simulink model "firefighting_drone_2"  (R2022b)
settings: Solver=FixedStepAuto  StartTime=0.0  StopTime=80  FixedStep=0.1  RelTol=1e-3
(part 3 of 4)

== system firefighting_drone_2/Search for Fire/Seaerch-fire/Search5/Move Arm1 ==
  Speed : Inport
  Starting Angle : Inport  Port=2
  Desired Angle : Inport  Port=3
  If : If
  If Action Subsystem : Subsystem  TreatAsAtomicUnit=on
  If Action Subsystem1 : Subsystem  TreatAsAtomicUnit=on
  Integrator1 : Integrator
  Scope : Scope
  Scope1 : Scope
  Subsystem : Subsystem
  Sum1 : Sum  Inputs=|++
  Sum2 : Sum  Inputs=|+-
  Sum3 : Sum  Inputs=|-+
  Switch : Switch  Criteria=u2 ~= 0  SaturateOnIntegerOverflow=off  InputSameDT=off
  Out1 : Outport  VectorParamsAs1DForOutWhenUnconnected=off
  Done : Outport  Port=2  VectorParamsAs1DForOutWhenUnconnected=off
  wires:
  Speed/1 -> Integrator1/1
  If Action Subsystem/1(Out1) -> Switch/3
  Sum2/1 -> If/1
  If/2 -> If Action Subsystem1/Action
  Starting Angle/1 -> Sum2/2, Sum3/2, Sum1/2
  Desired Angle/1 -> Scope1/1, Subsystem/1(Desired Angle), Sum2/1
  If Action Subsystem1/1(Out1) -> Switch/1, Switch/2
  If/1 -> If Action Subsystem/Action
  Integrator1/1 -> Sum1/1, Sum3/1
  Sum3/1 -> If Action Subsystem1/1(In1)
  Sum1/1 -> If Action Subsystem/1(In1)
  Switch/1 -> Subsystem/2(Current Angle)
  Subsystem/1(Out1) -> Scope/1, Out1/1
  Subsystem/2(Done) -> Done/1

== system firefighting_drone_2/Search for Fire/Seaerch-fire/Search5/Move Arm2 ==
  Speed : Inport
  Starting Angle : Inport  Port=2
  Desired Angle : Inport  Port=3
  If : If
  If Action Subsystem : Subsystem  TreatAsAtomicUnit=on
  If Action Subsystem1 : Subsystem  TreatAsAtomicUnit=on
  Integrator1 : Integrator
  Scope : Scope
  Subsystem : Subsystem
  Sum1 : Sum  Inputs=|++
  Sum2 : Sum  Inputs=|+-
  Sum3 : Sum  Inputs=|-+
  Switch : Switch  Criteria=u2 ~= 0  SaturateOnIntegerOverflow=off  InputSameDT=off
  Out1 : Outport  VectorParamsAs1DForOutWhenUnconnected=off
  Done : Outport  Port=2  VectorParamsAs1DForOutWhenUnconnected=off
  wires:
  Speed/1 -> Integrator1/1
  If Action Subsystem/1(Out1) -> Switch/3
  Sum2/1 -> If/1
  If/2 -> If Action Subsystem1/Action
  Starting Angle/1 -> Sum2/2, Sum3/2, Sum1/2
  Desired Angle/1 -> Subsystem/1(Desired Angle), Sum2/1
  If Action Subsystem1/1(Out1) -> Switch/1, Switch/2
  If/1 -> If Action Subsystem/Action
  Integrator1/1 -> Sum1/1, Sum3/1
  Sum3/1 -> If Action Subsystem1/1(In1)
  Sum1/1 -> If Action Subsystem/1(In1)
  Switch/1 -> Subsystem/2(Current Angle)
  Subsystem/1(Out1) -> Scope/1, Out1/1
  Subsystem/2(Done) -> Done/1

== system firefighting_drone_2/Search for Fire/Seaerch-fire/Search5/Move Arm3 ==
  Speed : Inport
  Starting Angle : Inport  Port=2
  Desired Angle : Inport  Port=3
  If : If
  If Action Subsystem : Subsystem  TreatAsAtomicUnit=on
  If Action Subsystem1 : Subsystem  TreatAsAtomicUnit=on
  Integrator1 : Integrator
  Scope : Scope
  Subsystem : Subsystem
  Sum1 : Sum  Inputs=|++
  Sum2 : Sum  Inputs=|+-
  Sum3 : Sum  Inputs=|-+
  Switch : Switch  Criteria=u2 ~= 0  SaturateOnIntegerOverflow=off  InputSameDT=off
  Out1 : Outport  VectorParamsAs1DForOutWhenUnconnected=off
  Done : Outport  Port=2  VectorParamsAs1DForOutWhenUnconnected=off
  wires:
  Speed/1 -> Integrator1/1
  If Action Subsystem/1(Out1) -> Switch/3
  Sum2/1 -> If/1
  If/2 -> If Action Subsystem1/Action
  Starting Angle/1 -> Sum2/2, Sum3/2, Sum1/2
  Desired Angle/1 -> Subsystem/1(Desired Angle), Sum2/1
  If Action Subsystem1/1(Out1) -> Switch/1, Switch/2
  If/1 -> If Action Subsystem/Action
  Integrator1/1 -> Sum1/1, Sum3/1
  Sum3/1 -> If Action Subsystem1/1(In1)
  Sum1/1 -> If Action Subsystem/1(In1)
  Switch/1 -> Subsystem/2(Current Angle)
  Subsystem/1(Out1) -> Scope/1, Out1/1
  Subsystem/2(Done) -> Done/1

== system firefighting_drone_2/Search for Fire/Seaerch-fire/Search6/Move Arm1 ==
  Speed : Inport
  Starting Angle : Inport  Port=2
  Desired Angle : Inport  Port=3
  If : If
  If Action Subsystem : Subsystem  TreatAsAtomicUnit=on
  If Action Subsystem1 : Subsystem  TreatAsAtomicUnit=on
  Integrator1 : Integrator
  Scope : Scope
  Scope1 : Scope
  Subsystem : Subsystem
  Sum1 : Sum  Inputs=|++
  Sum2 : Sum  Inputs=|+-
  Sum3 : Sum  Inputs=|-+
  Switch : Switch  Criteria=u2 ~= 0  SaturateOnIntegerOverflow=off  InputSameDT=off
  Out1 : Outport  VectorParamsAs1DForOutWhenUnconnected=off
  Done : Outport  Port=2  VectorParamsAs1DForOutWhenUnconnected=off
  wires:
  Speed/1 -> Integrator1/1
  If Action Subsystem/1(Out1) -> Switch/3
  Sum2/1 -> If/1
  If/2 -> If Action Subsystem1/Action
  Starting Angle/1 -> Sum2/2, Sum3/2, Sum1/2
  Desired Angle/1 -> Scope1/1, Subsystem/1(Desired Angle), Sum2/1
  If Action Subsystem1/1(Out1) -> Switch/1, Switch/2
  If/1 -> If Action Subsystem/Action
  Integrator1/1 -> Sum1/1, Sum3/1
  Sum3/1 -> If Action Subsystem1/1(In1)
  Sum1/1 -> If Action Subsystem/1(In1)
  Switch/1 -> Subsystem/2(Current Angle)
  Subsystem/1(Out1) -> Scope/1, Out1/1
  Subsystem/2(Done) -> Done/1

== system firefighting_drone_2/Search for Fire/Seaerch-fire/Search6/Move Arm2 ==
  Speed : Inport
  Starting Angle : Inport  Port=2
  Desired Angle : Inport  Port=3
  If : If
  If Action Subsystem : Subsystem  TreatAsAtomicUnit=on
  If Action Subsystem1 : Subsystem  TreatAsAtomicUnit=on
  Integrator1 : Integrator
  Scope : Scope
  Subsystem : Subsystem
  Sum1 : Sum  Inputs=|++
  Sum2 : Sum  Inputs=|+-
  Sum3 : Sum  Inputs=|-+
  Switch : Switch  Criteria=u2 ~= 0  SaturateOnIntegerOverflow=off  InputSameDT=off
  Out1 : Outport  VectorParamsAs1DForOutWhenUnconnected=off
  Done : Outport  Port=2  VectorParamsAs1DForOutWhenUnconnected=off
  wires:
  Speed/1 -> Integrator1/1
  If Action Subsystem/1(Out1) -> Switch/3
  Sum2/1 -> If/1
  If/2 -> If Action Subsystem1/Action
  Starting Angle/1 -> Sum2/2, Sum3/2, Sum1/2
  Desired Angle/1 -> Subsystem/1(Desired Angle), Sum2/1
  If Action Subsystem1/1(Out1) -> Switch/1, Switch/2
  If/1 -> If Action Subsystem/Action
  Integrator1/1 -> Sum1/1, Sum3/1
  Sum3/1 -> If Action Subsystem1/1(In1)
  Sum1/1 -> If Action Subsystem/1(In1)
  Switch/1 -> Subsystem/2(Current Angle)
  Subsystem/1(Out1) -> Scope/1, Out1/1
  Subsystem/2(Done) -> Done/1

== system firefighting_drone_2/Search for Fire/Seaerch-fire/Search6/Move Arm3 ==
  Speed : Inport
  Starting Angle : Inport  Port=2
  Desired Angle : Inport  Port=3
  If : If
  If Action Subsystem : Subsystem  TreatAsAtomicUnit=on
  If Action Subsystem1 : Subsystem  TreatAsAtomicUnit=on
  Integrator1 : Integrator
  Scope : Scope
  Subsystem : Subsystem
  Sum1 : Sum  Inputs=|++
  Sum2 : Sum  Inputs=|+-
  Sum3 : Sum  Inputs=|-+
  Switch : Switch  Criteria=u2 ~= 0  SaturateOnIntegerOverflow=off  InputSameDT=off
  Out1 : Outport  VectorParamsAs1DForOutWhenUnconnected=off
  Done : Outport  Port=2  VectorParamsAs1DForOutWhenUnconnected=off
  wires:
  Speed/1 -> Integrator1/1
  If Action Subsystem/1(Out1) -> Switch/3
  Sum2/1 -> If/1
  If/2 -> If Action Subsystem1/Action
  Starting Angle/1 -> Sum2/2, Sum3/2, Sum1/2
  Desired Angle/1 -> Subsystem/1(Desired Angle), Sum2/1
  If Action Subsystem1/1(Out1) -> Switch/1, Switch/2
  If/1 -> If Action Subsystem/Action
  Integrator1/1 -> Sum1/1, Sum3/1
  Sum3/1 -> If Action Subsystem1/1(In1)
  Sum1/1 -> If Action Subsystem/1(In1)
  Switch/1 -> Subsystem/2(Current Angle)
  Subsystem/1(Out1) -> Scope/1, Out1/1
  Subsystem/2(Done) -> Done/1

== system firefighting_drone_2/Search for Fire/Seaerch-fire/Search7/Move Arm1 ==
  Speed : Inport
  Starting Angle : Inport  Port=2
  Desired Angle : Inport  Port=3
  If : If
  If Action Subsystem : Subsystem  TreatAsAtomicUnit=on
  If Action Subsystem1 : Subsystem  TreatAsAtomicUnit=on
  Integrator1 : Integrator
  Scope : Scope
  Scope1 : Scope
  Subsystem : Subsystem
  Sum1 : Sum  Inputs=|++
  Sum2 : Sum  Inputs=|+-
  Sum3 : Sum  Inputs=|-+
  Switch : Switch  Criteria=u2 ~= 0  SaturateOnIntegerOverflow=off  InputSameDT=off
  Out1 : Outport  VectorParamsAs1DForOutWhenUnconnected=off
  Done : Outport  Port=2  VectorParamsAs1DForOutWhenUnconnected=off
  wires:
  Speed/1 -> Integrator1/1
  If Action Subsystem/1(Out1) -> Switch/3
  Sum2/1 -> If/1
  If/2 -> If Action Subsystem1/Action
  Starting Angle/1 -> Sum2/2, Sum3/2, Sum1/2
  Desired Angle/1 -> Scope1/1, Subsystem/1(Desired Angle), Sum2/1
  If Action Subsystem1/1(Out1) -> Switch/1, Switch/2
  If/1 -> If Action Subsystem/Action
  Integrator1/1 -> Sum1/1, Sum3/1
  Sum3/1 -> If Action Subsystem1/1(In1)
  Sum1/1 -> If Action Subsystem/1(In1)
  Switch/1 -> Subsystem/2(Current Angle)
  Subsystem/1(Out1) -> Scope/1, Out1/1
  Subsystem/2(Done) -> Done/1

== system firefighting_drone_2/Search for Fire/Seaerch-fire/Search7/Move Arm2 ==
  Speed : Inport
  Starting Angle : Inport  Port=2
  Desired Angle : Inport  Port=3
  If : If
  If Action Subsystem : Subsystem  TreatAsAtomicUnit=on
  If Action Subsystem1 : Subsystem  TreatAsAtomicUnit=on
  Integrator1 : Integrator
  Scope : Scope
  Subsystem : Subsystem
  Sum1 : Sum  Inputs=|++
  Sum2 : Sum  Inputs=|+-
  Sum3 : Sum  Inputs=|-+
  Switch : Switch  Criteria=u2 ~= 0  SaturateOnIntegerOverflow=off  InputSameDT=off
  Out1 : Outport  VectorParamsAs1DForOutWhenUnconnected=off
  Done : Outport  Port=2  VectorParamsAs1DForOutWhenUnconnected=off
  wires:
  Speed/1 -> Integrator1/1
  If Action Subsystem/1(Out1) -> Switch/3
  Sum2/1 -> If/1
  If/2 -> If Action Subsystem1/Action
  Starting Angle/1 -> Sum2/2, Sum3/2, Sum1/2
  Desired Angle/1 -> Subsystem/1(Desired Angle), Sum2/1
  If Action Subsystem1/1(Out1) -> Switch/1, Switch/2
  If/1 -> If Action Subsystem/Action
  Integrator1/1 -> Sum1/1, Sum3/1
  Sum3/1 -> If Action Subsystem1/1(In1)
  Sum1/1 -> If Action Subsystem/1(In1)
  Switch/1 -> Subsystem/2(Current Angle)
  Subsystem/1(Out1) -> Scope/1, Out1/1
  Subsystem/2(Done) -> Done/1

== system firefighting_drone_2/Search for Fire/Seaerch-fire/Search7/Move Arm3 ==
  Speed : Inport
  Starting Angle : Inport  Port=2
  Desired Angle : Inport  Port=3
  If : If
  If Action Subsystem : Subsystem  TreatAsAtomicUnit=on
  If Action Subsystem1 : Subsystem  TreatAsAtomicUnit=on
  Integrator1 : Integrator
  Scope : Scope
  Subsystem : Subsystem
  Sum1 : Sum  Inputs=|++
  Sum2 : Sum  Inputs=|+-
  Sum3 : Sum  Inputs=|-+
  Switch : Switch  Criteria=u2 ~= 0  SaturateOnIntegerOverflow=off  InputSameDT=off
  Out1 : Outport  VectorParamsAs1DForOutWhenUnconnected=off
  Done : Outport  Port=2  VectorParamsAs1DForOutWhenUnconnected=off
  wires:
  Speed/1 -> Integrator1/1
  If Action Subsystem/1(Out1) -> Switch/3
  Sum2/1 -> If/1
  If/2 -> If Action Subsystem1/Action
  Starting Angle/1 -> Sum2/2, Sum3/2, Sum1/2
  Desired Angle/1 -> Subsystem/1(Desired Angle), Sum2/1
  If Action Subsystem1/1(Out1) -> Switch/1, Switch/2
  If/1 -> If Action Subsystem/Action
  Integrator1/1 -> Sum1/1, Sum3/1
  Sum3/1 -> If Action Subsystem1/1(In1)
  Sum1/1 -> If Action Subsystem/1(In1)
  Switch/1 -> Subsystem/2(Current Angle)
  Subsystem/1(Out1) -> Scope/1, Out1/1
  Subsystem/2(Done) -> Done/1

== system firefighting_drone_2/Search for Fire/Seaerch-fire/Search8/Move Arm1 ==
  Speed : Inport
  Starting Angle : Inport  Port=2
  Desired Angle : Inport  Port=3
  If : If
  If Action Subsystem : Subsystem  TreatAsAtomicUnit=on
  If Action Subsystem1 : Subsystem  TreatAsAtomicUnit=on
  Integrator1 : Integrator
  Scope : Scope
  Scope1 : Scope
  Subsystem : Subsystem
  Sum1 : Sum  Inputs=|++
  Sum2 : Sum  Inputs=|+-
  Sum3 : Sum  Inputs=|-+
  Switch : Switch  Criteria=u2 ~= 0  SaturateOnIntegerOverflow=off  InputSameDT=off
  Out1 : Outport  VectorParamsAs1DForOutWhenUnconnected=off
  Done : Outport  Port=2  VectorParamsAs1DForOutWhenUnconnected=off
  wires:
  Speed/1 -> Integrator1/1
  If Action Subsystem/1(Out1) -> Switch/3
  Sum2/1 -> If/1
  If/2 -> If Action Subsystem1/Action
  Starting Angle/1 -> Sum2/2, Sum3/2, Sum1/2
  Desired Angle/1 -> Scope1/1, Subsystem/1(Desired Angle), Sum2/1
  If Action Subsystem1/1(Out1) -> Switch/1, Switch/2
  If/1 -> If Action Subsystem/Action
  Integrator1/1 -> Sum1/1, Sum3/1
  Sum3/1 -> If Action Subsystem1/1(In1)
  Sum1/1 -> If Action Subsystem/1(In1)
  Switch/1 -> Subsystem/2(Current Angle)
  Subsystem/1(Out1) -> Scope/1, Out1/1
  Subsystem/2(Done) -> Done/1

== system firefighting_drone_2/Search for Fire/Seaerch-fire/Search8/Move Arm2 ==
  Speed : Inport
  Starting Angle : Inport  Port=2
  Desired Angle : Inport  Port=3
  If : If
  If Action Subsystem : Subsystem  TreatAsAtomicUnit=on
  If Action Subsystem1 : Subsystem  TreatAsAtomicUnit=on
  Integrator1 : Integrator
  Scope : Scope
  Subsystem : Subsystem
  Sum1 : Sum  Inputs=|++
  Sum2 : Sum  Inputs=|+-
  Sum3 : Sum  Inputs=|-+
  Switch : Switch  Criteria=u2 ~= 0  SaturateOnIntegerOverflow=off  InputSameDT=off
  Out1 : Outport  VectorParamsAs1DForOutWhenUnconnected=off
  Done : Outport  Port=2  VectorParamsAs1DForOutWhenUnconnected=off
  wires:
  Speed/1 -> Integrator1/1
  If Action Subsystem/1(Out1) -> Switch/3
  Sum2/1 -> If/1
  If/2 -> If Action Subsystem1/Action
  Starting Angle/1 -> Sum2/2, Sum3/2, Sum1/2
  Desired Angle/1 -> Subsystem/1(Desired Angle), Sum2/1
  If Action Subsystem1/1(Out1) -> Switch/1, Switch/2
  If/1 -> If Action Subsystem/Action
  Integrator1/1 -> Sum1/1, Sum3/1
  Sum3/1 -> If Action Subsystem1/1(In1)
  Sum1/1 -> If Action Subsystem/1(In1)
  Switch/1 -> Subsystem/2(Current Angle)
  Subsystem/1(Out1) -> Scope/1, Out1/1
  Subsystem/2(Done) -> Done/1

== system firefighting_drone_2/Search for Fire/Seaerch-fire/Search8/Move Arm3 ==
  Speed : Inport
  Starting Angle : Inport  Port=2
  Desired Angle : Inport  Port=3
  If : If
  If Action Subsystem : Subsystem  TreatAsAtomicUnit=on
  If Action Subsystem1 : Subsystem  TreatAsAtomicUnit=on
  Integrator1 : Integrator
  Scope : Scope
  Subsystem : Subsystem
  Sum1 : Sum  Inputs=|++
  Sum2 : Sum  Inputs=|+-
  Sum3 : Sum  Inputs=|-+
  Switch : Switch  Criteria=u2 ~= 0  SaturateOnIntegerOverflow=off  InputSameDT=off
  Out1 : Outport  VectorParamsAs1DForOutWhenUnconnected=off
  Done : Outport  Port=2  VectorParamsAs1DForOutWhenUnconnected=off
  wires:
  Speed/1 -> Integrator1/1
  If Action Subsystem/1(Out1) -> Switch/3
  Sum2/1 -> If/1
  If/2 -> If Action Subsystem1/Action
  Starting Angle/1 -> Sum2/2, Sum3/2, Sum1/2
  Desired Angle/1 -> Subsystem/1(Desired Angle), Sum2/1
  If Action Subsystem1/1(Out1) -> Switch/1, Switch/2
  If/1 -> If Action Subsystem/Action
  Integrator1/1 -> Sum1/1, Sum3/1
  Sum3/1 -> If Action Subsystem1/1(In1)
  Sum1/1 -> If Action Subsystem/1(In1)
  Switch/1 -> Subsystem/2(Current Angle)
  Subsystem/1(Out1) -> Scope/1, Out1/1
  Subsystem/2(Done) -> Done/1

== system firefighting_drone_2/Search for Fire/Seaerch-fire/Search9/Move Arm1 ==
  Speed : Inport
  Starting Angle : Inport  Port=2
  Desired Angle : Inport  Port=3
  If : If
  If Action Subsystem : Subsystem  TreatAsAtomicUnit=on
  If Action Subsystem1 : Subsystem  TreatAsAtomicUnit=on
  Integrator1 : Integrator
  Scope : Scope
  Scope1 : Scope
  Subsystem : Subsystem
  Sum1 : Sum  Inputs=|++
  Sum2 : Sum  Inputs=|+-
  Sum3 : Sum  Inputs=|-+
  Switch : Switch  Criteria=u2 ~= 0  SaturateOnIntegerOverflow=off  InputSameDT=off
  Out1 : Outport  VectorParamsAs1DForOutWhenUnconnected=off
  Done : Outport  Port=2  VectorParamsAs1DForOutWhenUnconnected=off
  wires:
  Speed/1 -> Integrator1/1
  If Action Subsystem/1(Out1) -> Switch/3
  Sum2/1 -> If/1
  If/2 -> If Action Subsystem1/Action
  Starting Angle/1 -> Sum2/2, Sum3/2, Sum1/2
  Desired Angle/1 -> Scope1/1, Subsystem/1(Desired Angle), Sum2/1
  If Action Subsystem1/1(Out1) -> Switch/1, Switch/2
  If/1 -> If Action Subsystem/Action
  Integrator1/1 -> Sum1/1, Sum3/1
  Sum3/1 -> If Action Subsystem1/1(In1)
  Sum1/1 -> If Action Subsystem/1(In1)
  Switch/1 -> Subsystem/2(Current Angle)
  Subsystem/1(Out1) -> Scope/1, Out1/1
  Subsystem/2(Done) -> Done/1

== system firefighting_drone_2/Search for Fire/Seaerch-fire/Search9/Move Arm2 ==
  Speed : Inport
  Starting Angle : Inport  Port=2
  Desired Angle : Inport  Port=3
  If : If
  If Action Subsystem : Subsystem  TreatAsAtomicUnit=on
  If Action Subsystem1 : Subsystem  TreatAsAtomicUnit=on
  Integrator1 : Integrator
  Scope : Scope
  Subsystem : Subsystem
  Sum1 : Sum  Inputs=|++
  Sum2 : Sum  Inputs=|+-
  Sum3 : Sum  Inputs=|-+
  Switch : Switch  Criteria=u2 ~= 0  SaturateOnIntegerOverflow=off  InputSameDT=off
  Out1 : Outport  VectorParamsAs1DForOutWhenUnconnected=off
  Done : Outport  Port=2  VectorParamsAs1DForOutWhenUnconnected=off
  wires:
  Speed/1 -> Integrator1/1
  If Action Subsystem/1(Out1) -> Switch/3
  Sum2/1 -> If/1
  If/2 -> If Action Subsystem1/Action
  Starting Angle/1 -> Sum2/2, Sum3/2, Sum1/2
  Desired Angle/1 -> Subsystem/1(Desired Angle), Sum2/1
  If Action Subsystem1/1(Out1) -> Switch/1, Switch/2
  If/1 -> If Action Subsystem/Action
  Integrator1/1 -> Sum1/1, Sum3/1
  Sum3/1 -> If Action Subsystem1/1(In1)
  Sum1/1 -> If Action Subsystem/1(In1)
  Switch/1 -> Subsystem/2(Current Angle)
  Subsystem/1(Out1) -> Scope/1, Out1/1
  Subsystem/2(Done) -> Done/1

== system firefighting_drone_2/Search for Fire/Seaerch-fire/Search9/Move Arm3 ==
  Speed : Inport
  Starting Angle : Inport  Port=2
  Desired Angle : Inport  Port=3
  If : If
  If Action Subsystem : Subsystem  TreatAsAtomicUnit=on
  If Action Subsystem1 : Subsystem  TreatAsAtomicUnit=on
  Integrator1 : Integrator
  Scope : Scope
  Subsystem : Subsystem
  Sum1 : Sum  Inputs=|++
  Sum2 : Sum  Inputs=|+-
  Sum3 : Sum  Inputs=|-+
  Switch : Switch  Criteria=u2 ~= 0  SaturateOnIntegerOverflow=off  InputSameDT=off
  Out1 : Outport  VectorParamsAs1DForOutWhenUnconnected=off
  Done : Outport  Port=2  VectorParamsAs1DForOutWhenUnconnected=off
  wires:
  Speed/1 -> Integrator1/1
  If Action Subsystem/1(Out1) -> Switch/3
  Sum2/1 -> If/1
  If/2 -> If Action Subsystem1/Action
  Starting Angle/1 -> Sum2/2, Sum3/2, Sum1/2
  Desired Angle/1 -> Subsystem/1(Desired Angle), Sum2/1
  If Action Subsystem1/1(Out1) -> Switch/1, Switch/2
  If/1 -> If Action Subsystem/Action
  Integrator1/1 -> Sum1/1, Sum3/1
  Sum3/1 -> If Action Subsystem1/1(In1)
  Sum1/1 -> If Action Subsystem/1(In1)
  Switch/1 -> Subsystem/2(Current Angle)
  Subsystem/1(Out1) -> Scope/1, Out1/1
  Subsystem/2(Done) -> Done/1

== system firefighting_drone_2/Search for Fire/Seaerch-fire/Search/Move Arm1/If Action Subsystem ==
  In1 : Inport
  Action Port : ActionPort  ActionPortLabel=if(u1 > 0)
  Out1 : Outport  VectorParamsAs1DForOutWhenUnconnected=off
  wires:
  In1/1 -> Out1/1

== system firefighting_drone_2/Search for Fire/Seaerch-fire/Search/Move Arm1/If Action Subsystem1 ==
  In1 : Inport
  Action Port : ActionPort  ActionPortLabel=else
  Out1 : Outport  VectorParamsAs1DForOutWhenUnconnected=off
  wires:
  In1/1 -> Out1/1

== system firefighting_drone_2/Search for Fire/Seaerch-fire/Search/Move Arm1/Subsystem ==
  Desired Angle : Inport
  Current Angle : Inport  Port=2
  Abs : Abs  SaturateOnIntegerOverflow=off
  Constant : Constant
  Logical Operator : Logic  Operator=OR  AllPortsSameDT=off  OutDataTypeStr=boolean
  Memory : Memory
  Relational Operator : RelationalOperator  Operator=<=  OutDataTypeStr=boolean  RndMeth=Simplest  InputSameDT=off
  Sum : Sum  Inputs=|+-
  Switch1 : Switch  Criteria=u2 > Threshold  SaturateOnIntegerOverflow=off  InputSameDT=off
  Out1 : Outport  VectorParamsAs1DForOutWhenUnconnected=off
  Done : Outport  Port=2  VectorParamsAs1DForOutWhenUnconnected=off
  wires:
  Switch1/1 -> Out1/1
  Desired Angle/1 -> Sum/1, Switch1/1
  Current Angle/1 -> Switch1/3, Sum/2
  Sum/1 -> Abs/1
  Abs/1 -> Relational Operator/1
  Constant/1 -> Relational Operator/2
  Relational Operator/1 -> Logical Operator/2
  Logical Operator/1 -> Memory/1, Done/1, Switch1/2
  Memory/1 -> Logical Operator/1

== system firefighting_drone_2/Search for Fire/Seaerch-fire/Search/Move Arm2/If Action Subsystem ==
  In1 : Inport
  Action Port : ActionPort  ActionPortLabel=if(u1 > 0)
  Out1 : Outport  VectorParamsAs1DForOutWhenUnconnected=off
  wires:
  In1/1 -> Out1/1

== system firefighting_drone_2/Search for Fire/Seaerch-fire/Search/Move Arm2/If Action Subsystem1 ==
  In1 : Inport
  Action Port : ActionPort  ActionPortLabel=else
  Out1 : Outport  VectorParamsAs1DForOutWhenUnconnected=off
  wires:
  In1/1 -> Out1/1

== system firefighting_drone_2/Search for Fire/Seaerch-fire/Search/Move Arm2/Subsystem ==
  Desired Angle : Inport
  Current Angle : Inport  Port=2
  Abs : Abs  SaturateOnIntegerOverflow=off
  Constant : Constant
  Logical Operator : Logic  Operator=OR  AllPortsSameDT=off  OutDataTypeStr=boolean
  Memory : Memory
  Relational Operator : RelationalOperator  Operator=<=  OutDataTypeStr=boolean  RndMeth=Simplest  InputSameDT=off
  Sum : Sum  Inputs=|+-
  Switch1 : Switch  Criteria=u2 > Threshold  SaturateOnIntegerOverflow=off  InputSameDT=off
  Out1 : Outport  VectorParamsAs1DForOutWhenUnconnected=off
  Done : Outport  Port=2  VectorParamsAs1DForOutWhenUnconnected=off
  wires:
  Switch1/1 -> Out1/1
  Desired Angle/1 -> Sum/1, Switch1/1
  Current Angle/1 -> Switch1/3, Sum/2
  Sum/1 -> Abs/1
  Abs/1 -> Relational Operator/1
  Constant/1 -> Relational Operator/2
  Relational Operator/1 -> Logical Operator/2
  Logical Operator/1 -> Memory/1, Done/1, Switch1/2
  Memory/1 -> Logical Operator/1

== system firefighting_drone_2/Search for Fire/Seaerch-fire/Search/Move Arm3/If Action Subsystem ==
  In1 : Inport
  Action Port : ActionPort  ActionPortLabel=if(u1 > 0)
  Out1 : Outport  VectorParamsAs1DForOutWhenUnconnected=off
  wires:
  In1/1 -> Out1/1

== system firefighting_drone_2/Search for Fire/Seaerch-fire/Search/Move Arm3/If Action Subsystem1 ==
  In1 : Inport
  Action Port : ActionPort  ActionPortLabel=else
  Out1 : Outport  VectorParamsAs1DForOutWhenUnconnected=off
  wires:
  In1/1 -> Out1/1

== system firefighting_drone_2/Search for Fire/Seaerch-fire/Search/Move Arm3/Subsystem ==
  Desired Angle : Inport
  Current Angle : Inport  Port=2
  Abs : Abs  SaturateOnIntegerOverflow=off
  Constant : Constant
  Logical Operator : Logic  Operator=OR  AllPortsSameDT=off  OutDataTypeStr=boolean
  Memory : Memory
  Relational Operator : RelationalOperator  Operator=<=  OutDataTypeStr=boolean  RndMeth=Simplest  InputSameDT=off
  Sum : Sum  Inputs=|+-
  Switch1 : Switch  Criteria=u2 > Threshold  SaturateOnIntegerOverflow=off  InputSameDT=off
  Out1 : Outport  VectorParamsAs1DForOutWhenUnconnected=off
  Done : Outport  Port=2  VectorParamsAs1DForOutWhenUnconnected=off
  wires:
  Switch1/1 -> Out1/1
  Desired Angle/1 -> Sum/1, Switch1/1
  Current Angle/1 -> Switch1/3, Sum/2
  Sum/1 -> Abs/1
  Abs/1 -> Relational Operator/1
  Constant/1 -> Relational Operator/2
  Relational Operator/1 -> Logical Operator/2
  Logical Operator/1 -> Memory/1, Done/1, Switch1/2
  Memory/1 -> Logical Operator/1

== system firefighting_drone_2/Search for Fire/Seaerch-fire/Search1/Move Arm1/If Action Subsystem ==
  In1 : Inport
  Action Port : ActionPort  ActionPortLabel=if(u1 > 0)
  Out1 : Outport  VectorParamsAs1DForOutWhenUnconnected=off
  wires:
  In1/1 -> Out1/1

== system firefighting_drone_2/Search for Fire/Seaerch-fire/Search1/Move Arm1/If Action Subsystem1 ==
  In1 : Inport
  Action Port : ActionPort  ActionPortLabel=else
  Out1 : Outport  VectorParamsAs1DForOutWhenUnconnected=off
  wires:
  In1/1 -> Out1/1

== system firefighting_drone_2/Search for Fire/Seaerch-fire/Search1/Move Arm1/Subsystem ==
  Desired Angle : Inport
  Current Angle : Inport  Port=2
  Abs : Abs  SaturateOnIntegerOverflow=off
  Constant : Constant
  Logical Operator : Logic  Operator=OR  AllPortsSameDT=off  OutDataTypeStr=boolean
  Memory : Memory
  Relational Operator : RelationalOperator  Operator=<=  OutDataTypeStr=boolean  RndMeth=Simplest  InputSameDT=off
  Scope : Scope
  Scope1 : Scope
  Sum : Sum  Inputs=|+-
  Switch1 : Switch  Criteria=u2 > Threshold  SaturateOnIntegerOverflow=off  InputSameDT=off
  Out1 : Outport  VectorParamsAs1DForOutWhenUnconnected=off
  Done : Outport  Port=2  VectorParamsAs1DForOutWhenUnconnected=off
  wires:
  Switch1/1 -> Out1/1
  Desired Angle/1 -> Scope/1, Sum/1, Switch1/1
  Current Angle/1 -> Scope1/1, Switch1/3, Sum/2
  Sum/1 -> Abs/1
  Abs/1 -> Relational Operator/1
  Constant/1 -> Relational Operator/2
  Relational Operator/1 -> Logical Operator/2
  Logical Operator/1 -> Memory/1, Done/1, Switch1/2
  Memory/1 -> Logical Operator/1

== system firefighting_drone_2/Search for Fire/Seaerch-fire/Search1/Move Arm2/If Action Subsystem ==
  In1 : Inport
  Action Port : ActionPort  ActionPortLabel=if(u1 > 0)
  Out1 : Outport  VectorParamsAs1DForOutWhenUnconnected=off
  wires:
  In1/1 -> Out1/1

== system firefighting_drone_2/Search for Fire/Seaerch-fire/Search1/Move Arm2/If Action Subsystem1 ==
  In1 : Inport
  Action Port : ActionPort  ActionPortLabel=else
  Out1 : Outport  VectorParamsAs1DForOutWhenUnconnected=off
  wires:
  In1/1 -> Out1/1

== system firefighting_drone_2/Search for Fire/Seaerch-fire/Search1/Move Arm2/Subsystem ==
  Desired Angle : Inport
  Current Angle : Inport  Port=2
  Abs : Abs  SaturateOnIntegerOverflow=off
  Constant : Constant
  Logical Operator : Logic  Operator=OR  AllPortsSameDT=off  OutDataTypeStr=boolean
  Memory : Memory
  Relational Operator : RelationalOperator  Operator=<=  OutDataTypeStr=boolean  RndMeth=Simplest  InputSameDT=off
  Sum : Sum  Inputs=|+-
  Switch1 : Switch  Criteria=u2 > Threshold  SaturateOnIntegerOverflow=off  InputSameDT=off
  Out1 : Outport  VectorParamsAs1DForOutWhenUnconnected=off
  Done : Outport  Port=2  VectorParamsAs1DForOutWhenUnconnected=off
  wires:
  Switch1/1 -> Out1/1
  Desired Angle/1 -> Sum/1, Switch1/1
  Current Angle/1 -> Switch1/3, Sum/2
  Sum/1 -> Abs/1
  Abs/1 -> Relational Operator/1
  Constant/1 -> Relational Operator/2
  Relational Operator/1 -> Logical Operator/2
  Logical Operator/1 -> Memory/1, Done/1, Switch1/2
  Memory/1 -> Logical Operator/1

== system firefighting_drone_2/Search for Fire/Seaerch-fire/Search1/Move Arm3/If Action Subsystem ==
  In1 : Inport
  Action Port : ActionPort  ActionPortLabel=if(u1 > 0)
  Out1 : Outport  VectorParamsAs1DForOutWhenUnconnected=off
  wires:
  In1/1 -> Out1/1

== system firefighting_drone_2/Search for Fire/Seaerch-fire/Search1/Move Arm3/If Action Subsystem1 ==
  In1 : Inport
  Action Port : ActionPort  ActionPortLabel=else
  Out1 : Outport  VectorParamsAs1DForOutWhenUnconnected=off
  wires:
  In1/1 -> Out1/1

== system firefighting_drone_2/Search for Fire/Seaerch-fire/Search1/Move Arm3/Subsystem ==
  Desired Angle : Inport
  Current Angle : Inport  Port=2
  Abs : Abs  SaturateOnIntegerOverflow=off
  Constant : Constant
  Logical Operator : Logic  Operator=OR  AllPortsSameDT=off  OutDataTypeStr=boolean
  Memory : Memory
  Relational Operator : RelationalOperator  Operator=<=  OutDataTypeStr=boolean  RndMeth=Simplest  InputSameDT=off
  Sum : Sum  Inputs=|+-
  Switch1 : Switch  Criteria=u2 > Threshold  SaturateOnIntegerOverflow=off  InputSameDT=off
  Out1 : Outport  VectorParamsAs1DForOutWhenUnconnected=off
  Done : Outport  Port=2  VectorParamsAs1DForOutWhenUnconnected=off
  wires:
  Switch1/1 -> Out1/1
  Desired Angle/1 -> Sum/1, Switch1/1
  Current Angle/1 -> Switch1/3, Sum/2
  Sum/1 -> Abs/1
  Abs/1 -> Relational Operator/1
  Constant/1 -> Relational Operator/2
  Relational Operator/1 -> Logical Operator/2
  Logical Operator/1 -> Memory/1, Done/1, Switch1/2
  Memory/1 -> Logical Operator/1

== system firefighting_drone_2/Search for Fire/Seaerch-fire/Search10/Move Arm1/If Action Subsystem ==
  In1 : Inport
  Action Port : ActionPort  ActionPortLabel=if(u1 > 0)
  Out1 : Outport  VectorParamsAs1DForOutWhenUnconnected=off
  wires:
  In1/1 -> Out1/1

== system firefighting_drone_2/Search for Fire/Seaerch-fire/Search10/Move Arm1/If Action Subsystem1 ==
  In1 : Inport
  Action Port : ActionPort  ActionPortLabel=else
  Out1 : Outport  VectorParamsAs1DForOutWhenUnconnected=off
  wires:
  In1/1 -> Out1/1

== system firefighting_drone_2/Search for Fire/Seaerch-fire/Search10/Move Arm1/Subsystem ==
  Desired Angle : Inport
  Current Angle : Inport  Port=2
  Abs : Abs  SaturateOnIntegerOverflow=off
  Constant : Constant
  Logical Operator : Logic  Operator=OR  AllPortsSameDT=off  OutDataTypeStr=boolean
  Memory : Memory
  Relational Operator : RelationalOperator  Operator=<=  OutDataTypeStr=boolean  RndMeth=Simplest  InputSameDT=off
  Scope : Scope
  Scope1 : Scope
  Sum : Sum  Inputs=|+-
  Switch1 : Switch  Criteria=u2 > Threshold  SaturateOnIntegerOverflow=off  InputSameDT=off
  Out1 : Outport  VectorParamsAs1DForOutWhenUnconnected=off
  Done : Outport  Port=2  VectorParamsAs1DForOutWhenUnconnected=off
  wires:
  Switch1/1 -> Out1/1
  Desired Angle/1 -> Scope/1, Sum/1, Switch1/1
  Current Angle/1 -> Scope1/1, Switch1/3, Sum/2
  Sum/1 -> Abs/1
  Abs/1 -> Relational Operator/1
  Constant/1 -> Relational Operator/2
  Relational Operator/1 -> Logical Operator/2
  Logical Operator/1 -> Memory/1, Done/1, Switch1/2
  Memory/1 -> Logical Operator/1

== system firefighting_drone_2/Search for Fire/Seaerch-fire/Search10/Move Arm2/If Action Subsystem ==
  In1 : Inport
  Action Port : ActionPort  ActionPortLabel=if(u1 > 0)
  Out1 : Outport  VectorParamsAs1DForOutWhenUnconnected=off
  wires:
  In1/1 -> Out1/1

== system firefighting_drone_2/Search for Fire/Seaerch-fire/Search10/Move Arm2/If Action Subsystem1 ==
  In1 : Inport
  Action Port : ActionPort  ActionPortLabel=else
  Out1 : Outport  VectorParamsAs1DForOutWhenUnconnected=off
  wires:
  In1/1 -> Out1/1

== system firefighting_drone_2/Search for Fire/Seaerch-fire/Search10/Move Arm2/Subsystem ==
  Desired Angle : Inport
  Current Angle : Inport  Port=2
  Abs : Abs  SaturateOnIntegerOverflow=off
  Constant : Constant
  Logical Operator : Logic  Operator=OR  AllPortsSameDT=off  OutDataTypeStr=boolean
  Memory : Memory
  Relational Operator : RelationalOperator  Operator=<=  OutDataTypeStr=boolean  RndMeth=Simplest  InputSameDT=off
  Sum : Sum  Inputs=|+-
  Switch1 : Switch  Criteria=u2 > Threshold  SaturateOnIntegerOverflow=off  InputSameDT=off
  Out1 : Outport  VectorParamsAs1DForOutWhenUnconnected=off
  Done : Outport  Port=2  VectorParamsAs1DForOutWhenUnconnected=off
  wires:
  Switch1/1 -> Out1/1
  Desired Angle/1 -> Sum/1, Switch1/1
  Current Angle/1 -> Switch1/3, Sum/2
  Sum/1 -> Abs/1
  Abs/1 -> Relational Operator/1
  Constant/1 -> Relational Operator/2
  Relational Operator/1 -> Logical Operator/2
  Logical Operator/1 -> Memory/1, Done/1, Switch1/2
  Memory/1 -> Logical Operator/1

== system firefighting_drone_2/Search for Fire/Seaerch-fire/Search10/Move Arm3/If Action Subsystem ==
  In1 : Inport
  Action Port : ActionPort  ActionPortLabel=if(u1 > 0)
  Out1 : Outport  VectorParamsAs1DForOutWhenUnconnected=off
  wires:
  In1/1 -> Out1/1

== system firefighting_drone_2/Search for Fire/Seaerch-fire/Search10/Move Arm3/If Action Subsystem1 ==
  In1 : Inport
  Action Port : ActionPort  ActionPortLabel=else
  Out1 : Outport  VectorParamsAs1DForOutWhenUnconnected=off
  wires:
  In1/1 -> Out1/1

== system firefighting_drone_2/Search for Fire/Seaerch-fire/Search10/Move Arm3/Subsystem ==
  Desired Angle : Inport
  Current Angle : Inport  Port=2
  Abs : Abs  SaturateOnIntegerOverflow=off
  Constant : Constant
  Logical Operator : Logic  Operator=OR  AllPortsSameDT=off  OutDataTypeStr=boolean
  Memory : Memory
  Relational Operator : RelationalOperator  Operator=<=  OutDataTypeStr=boolean  RndMeth=Simplest  InputSameDT=off
  Sum : Sum  Inputs=|+-
  Switch1 : Switch  Criteria=u2 > Threshold  SaturateOnIntegerOverflow=off  InputSameDT=off
  Out1 : Outport  VectorParamsAs1DForOutWhenUnconnected=off
  Done : Outport  Port=2  VectorParamsAs1DForOutWhenUnconnected=off
  wires:
  Switch1/1 -> Out1/1
  Desired Angle/1 -> Sum/1, Switch1/1
  Current Angle/1 -> Switch1/3, Sum/2
  Sum/1 -> Abs/1
  Abs/1 -> Relational Operator/1
  Constant/1 -> Relational Operator/2
  Relational Operator/1 -> Logical Operator/2
  Logical Operator/1 -> Memory/1, Done/1, Switch1/2
  Memory/1 -> Logical Operator/1

== system firefighting_drone_2/Search for Fire/Seaerch-fire/Search2/Move Arm1/If Action Subsystem ==
  In1 : Inport
  Action Port : ActionPort  ActionPortLabel=if(u1 > 0)
  Out1 : Outport  VectorParamsAs1DForOutWhenUnconnected=off
  wires:
  In1/1 -> Out1/1

== system firefighting_drone_2/Search for Fire/Seaerch-fire/Search2/Move Arm1/If Action Subsystem1 ==
  In1 : Inport
  Action Port : ActionPort  ActionPortLabel=else
  Out1 : Outport  VectorParamsAs1DForOutWhenUnconnected=off
  wires:
  In1/1 -> Out1/1

== system firefighting_drone_2/Search for Fire/Seaerch-fire/Search2/Move Arm1/Subsystem ==
  Desired Angle : Inport
  Current Angle : Inport  Port=2
  Abs : Abs  SaturateOnIntegerOverflow=off
  Constant : Constant
  Logical Operator : Logic  Operator=OR  AllPortsSameDT=off  OutDataTypeStr=boolean
  Memory : Memory
  Relational Operator : RelationalOperator  Operator=<=  OutDataTypeStr=boolean  RndMeth=Simplest  InputSameDT=off
  Scope : Scope
  Scope1 : Scope
  Sum : Sum  Inputs=|+-
  Switch1 : Switch  Criteria=u2 > Threshold  SaturateOnIntegerOverflow=off  InputSameDT=off
  Out1 : Outport  VectorParamsAs1DForOutWhenUnconnected=off
  Done : Outport  Port=2  VectorParamsAs1DForOutWhenUnconnected=off
  wires:
  Switch1/1 -> Out1/1
  Desired Angle/1 -> Scope/1, Sum/1, Switch1/1
  Current Angle/1 -> Scope1/1, Switch1/3, Sum/2
  Sum/1 -> Abs/1
  Abs/1 -> Relational Operator/1
  Constant/1 -> Relational Operator/2
  Relational Operator/1 -> Logical Operator/2
  Logical Operator/1 -> Memory/1, Done/1, Switch1/2
  Memory/1 -> Logical Operator/1

== system firefighting_drone_2/Search for Fire/Seaerch-fire/Search2/Move Arm2/If Action Subsystem ==
  In1 : Inport
  Action Port : ActionPort  ActionPortLabel=if(u1 > 0)
  Out1 : Outport  VectorParamsAs1DForOutWhenUnconnected=off
  wires:
  In1/1 -> Out1/1

== system firefighting_drone_2/Search for Fire/Seaerch-fire/Search2/Move Arm2/If Action Subsystem1 ==
  In1 : Inport
  Action Port : ActionPort  ActionPortLabel=else
  Out1 : Outport  VectorParamsAs1DForOutWhenUnconnected=off
  wires:
  In1/1 -> Out1/1

== system firefighting_drone_2/Search for Fire/Seaerch-fire/Search2/Move Arm2/Subsystem ==
  Desired Angle : Inport
  Current Angle : Inport  Port=2
  Abs : Abs  SaturateOnIntegerOverflow=off
  Constant : Constant
  Logical Operator : Logic  Operator=OR  AllPortsSameDT=off  OutDataTypeStr=boolean
  Memory : Memory
  Relational Operator : RelationalOperator  Operator=<=  OutDataTypeStr=boolean  RndMeth=Simplest  InputSameDT=off
  Sum : Sum  Inputs=|+-
  Switch1 : Switch  Criteria=u2 > Threshold  SaturateOnIntegerOverflow=off  InputSameDT=off
  Out1 : Outport  VectorParamsAs1DForOutWhenUnconnected=off
  Done : Outport  Port=2  VectorParamsAs1DForOutWhenUnconnected=off
  wires:
  Switch1/1 -> Out1/1
  Desired Angle/1 -> Sum/1, Switch1/1
  Current Angle/1 -> Switch1/3, Sum/2
  Sum/1 -> Abs/1
  Abs/1 -> Relational Operator/1
  Constant/1 -> Relational Operator/2
  Relational Operator/1 -> Logical Operator/2
  Logical Operator/1 -> Memory/1, Done/1, Switch1/2
  Memory/1 -> Logical Operator/1

== system firefighting_drone_2/Search for Fire/Seaerch-fire/Search2/Move Arm3/If Action Subsystem ==
  In1 : Inport
  Action Port : ActionPort  ActionPortLabel=if(u1 > 0)
  Out1 : Outport  VectorParamsAs1DForOutWhenUnconnected=off
  wires:
  In1/1 -> Out1/1

== system firefighting_drone_2/Search for Fire/Seaerch-fire/Search2/Move Arm3/If Action Subsystem1 ==
  In1 : Inport
  Action Port : ActionPort  ActionPortLabel=else
  Out1 : Outport  VectorParamsAs1DForOutWhenUnconnected=off
  wires:
  In1/1 -> Out1/1

== system firefighting_drone_2/Search for Fire/Seaerch-fire/Search2/Move Arm3/Subsystem ==
  Desired Angle : Inport
  Current Angle : Inport  Port=2
  Abs : Abs  SaturateOnIntegerOverflow=off
  Constant : Constant
  Logical Operator : Logic  Operator=OR  AllPortsSameDT=off  OutDataTypeStr=boolean
  Memory : Memory
  Relational Operator : RelationalOperator  Operator=<=  OutDataTypeStr=boolean  RndMeth=Simplest  InputSameDT=off
  Sum : Sum  Inputs=|+-
  Switch1 : Switch  Criteria=u2 > Threshold  SaturateOnIntegerOverflow=off  InputSameDT=off
  Out1 : Outport  VectorParamsAs1DForOutWhenUnconnected=off
  Done : Outport  Port=2  VectorParamsAs1DForOutWhenUnconnected=off
  wires:
  Switch1/1 -> Out1/1
  Desired Angle/1 -> Sum/1, Switch1/1
  Current Angle/1 -> Switch1/3, Sum/2
  Sum/1 -> Abs/1
  Abs/1 -> Relational Operator/1
  Constant/1 -> Relational Operator/2
  Relational Operator/1 -> Logical Operator/2
  Logical Operator/1 -> Memory/1, Done/1, Switch1/2
  Memory/1 -> Logical Operator/1

== system firefighting_drone_2/Search for Fire/Seaerch-fire/Search3/Move Arm1/If Action Subsystem ==
  In1 : Inport
  Action Port : ActionPort  ActionPortLabel=if(u1 > 0)
  Out1 : Outport  VectorParamsAs1DForOutWhenUnconnected=off
  wires:
  In1/1 -> Out1/1

== system firefighting_drone_2/Search for Fire/Seaerch-fire/Search3/Move Arm1/If Action Subsystem1 ==
  In1 : Inport
  Action Port : ActionPort  ActionPortLabel=else
  Out1 : Outport  VectorParamsAs1DForOutWhenUnconnected=off
  wires:
  In1/1 -> Out1/1

== system firefighting_drone_2/Search for Fire/Seaerch-fire/Search3/Move Arm1/Subsystem ==
  Desired Angle : Inport
  Current Angle : Inport  Port=2
  Abs : Abs  SaturateOnIntegerOverflow=off
  Constant : Constant
  Logical Operator : Logic  Operator=OR  AllPortsSameDT=off  OutDataTypeStr=boolean
  Memory : Memory
  Relational Operator : RelationalOperator  Operator=<=  OutDataTypeStr=boolean  RndMeth=Simplest  InputSameDT=off
  Scope : Scope
  Scope1 : Scope
  Sum : Sum  Inputs=|+-
  Switch1 : Switch  Criteria=u2 > Threshold  SaturateOnIntegerOverflow=off  InputSameDT=off
  Out1 : Outport  VectorParamsAs1DForOutWhenUnconnected=off
  Done : Outport  Port=2  VectorParamsAs1DForOutWhenUnconnected=off
  wires:
  Switch1/1 -> Out1/1
  Desired Angle/1 -> Scope/1, Sum/1, Switch1/1
  Current Angle/1 -> Scope1/1, Switch1/3, Sum/2
  Sum/1 -> Abs/1
  Abs/1 -> Relational Operator/1
  Constant/1 -> Relational Operator/2
  Relational Operator/1 -> Logical Operator/2
  Logical Operator/1 -> Memory/1, Done/1, Switch1/2
  Memory/1 -> Logical Operator/1

== system firefighting_drone_2/Search for Fire/Seaerch-fire/Search3/Move Arm2/If Action Subsystem ==
  In1 : Inport
  Action Port : ActionPort  ActionPortLabel=if(u1 > 0)
  Out1 : Outport  VectorParamsAs1DForOutWhenUnconnected=off
  wires:
  In1/1 -> Out1/1

== system firefighting_drone_2/Search for Fire/Seaerch-fire/Search3/Move Arm2/If Action Subsystem1 ==
  In1 : Inport
  Action Port : ActionPort  ActionPortLabel=else
  Out1 : Outport  VectorParamsAs1DForOutWhenUnconnected=off
  wires:
  In1/1 -> Out1/1

== system firefighting_drone_2/Search for Fire/Seaerch-fire/Search3/Move Arm2/Subsystem ==
  Desired Angle : Inport
  Current Angle : Inport  Port=2
  Abs : Abs  SaturateOnIntegerOverflow=off
  Constant : Constant
  Logical Operator : Logic  Operator=OR  AllPortsSameDT=off  OutDataTypeStr=boolean
  Memory : Memory
  Relational Operator : RelationalOperator  Operator=<=  OutDataTypeStr=boolean  RndMeth=Simplest  InputSameDT=off
  Sum : Sum  Inputs=|+-
  Switch1 : Switch  Criteria=u2 > Threshold  SaturateOnIntegerOverflow=off  InputSameDT=off
  Out1 : Outport  VectorParamsAs1DForOutWhenUnconnected=off
  Done : Outport  Port=2  VectorParamsAs1DForOutWhenUnconnected=off
  wires:
  Switch1/1 -> Out1/1
  Desired Angle/1 -> Sum/1, Switch1/1
  Current Angle/1 -> Switch1/3, Sum/2
  Sum/1 -> Abs/1
  Abs/1 -> Relational Operator/1
  Constant/1 -> Relational Operator/2
  Relational Operator/1 -> Logical Operator/2
  Logical Operator/1 -> Memory/1, Done/1, Switch1/2
  Memory/1 -> Logical Operator/1

== system firefighting_drone_2/Search for Fire/Seaerch-fire/Search3/Move Arm3/If Action Subsystem ==
  In1 : Inport
  Action Port : ActionPort  ActionPortLabel=if(u1 > 0)
  Out1 : Outport  VectorParamsAs1DForOutWhenUnconnected=off
  wires:
  In1/1 -> Out1/1

== system firefighting_drone_2/Search for Fire/Seaerch-fire/Search3/Move Arm3/If Action Subsystem1 ==
  In1 : Inport
  Action Port : ActionPort  ActionPortLabel=else
  Out1 : Outport  VectorParamsAs1DForOutWhenUnconnected=off
  wires:
  In1/1 -> Out1/1

== system firefighting_drone_2/Search for Fire/Seaerch-fire/Search3/Move Arm3/Subsystem ==
  Desired Angle : Inport
  Current Angle : Inport  Port=2
  Abs : Abs  SaturateOnIntegerOverflow=off
  Constant : Constant
  Logical Operator : Logic  Operator=OR  AllPortsSameDT=off  OutDataTypeStr=boolean
  Memory : Memory
  Relational Operator : RelationalOperator  Operator=<=  OutDataTypeStr=boolean  RndMeth=Simplest  InputSameDT=off
  Sum : Sum  Inputs=|+-
  Switch1 : Switch  Criteria=u2 > Threshold  SaturateOnIntegerOverflow=off  InputSameDT=off
  Out1 : Outport  VectorParamsAs1DForOutWhenUnconnected=off
  Done : Outport  Port=2  VectorParamsAs1DForOutWhenUnconnected=off
  wires:
  Switch1/1 -> Out1/1
  Desired Angle/1 -> Sum/1, Switch1/1
  Current Angle/1 -> Switch1/3, Sum/2
  Sum/1 -> Abs/1
  Abs/1 -> Relational Operator/1
  Constant/1 -> Relational Operator/2
  Relational Operator/1 -> Logical Operator/2
  Logical Operator/1 -> Memory/1, Done/1, Switch1/2
  Memory/1 -> Logical Operator/1

== system firefighting_drone_2/Search for Fire/Seaerch-fire/Search4/Move Arm1/If Action Subsystem ==
  In1 : Inport
  Action Port : ActionPort  ActionPortLabel=if(u1 > 0)
  Out1 : Outport  VectorParamsAs1DForOutWhenUnconnected=off
  wires:
  In1/1 -> Out1/1

== system firefighting_drone_2/Search for Fire/Seaerch-fire/Search4/Move Arm1/If Action Subsystem1 ==
  In1 : Inport
  Action Port : ActionPort  ActionPortLabel=else
  Out1 : Outport  VectorParamsAs1DForOutWhenUnconnected=off
  wires:
  In1/1 -> Out1/1

== system firefighting_drone_2/Search for Fire/Seaerch-fire/Search4/Move Arm1/Subsystem ==
  Desired Angle : Inport
  Current Angle : Inport  Port=2
  Abs : Abs  SaturateOnIntegerOverflow=off
  Constant : Constant
  Logical Operator : Logic  Operator=OR  AllPortsSameDT=off  OutDataTypeStr=boolean
  Memory : Memory
  Relational Operator : RelationalOperator  Operator=<=  OutDataTypeStr=boolean  RndMeth=Simplest  InputSameDT=off
  Scope : Scope
  Scope1 : Scope
  Sum : Sum  Inputs=|+-
  Switch1 : Switch  Criteria=u2 > Threshold  SaturateOnIntegerOverflow=off  InputSameDT=off
  Out1 : Outport  VectorParamsAs1DForOutWhenUnconnected=off
  Done : Outport  Port=2  VectorParamsAs1DForOutWhenUnconnected=off
  wires:
  Switch1/1 -> Out1/1
  Desired Angle/1 -> Scope/1, Sum/1, Switch1/1
  Current Angle/1 -> Scope1/1, Switch1/3, Sum/2
  Sum/1 -> Abs/1
  Abs/1 -> Relational Operator/1
  Constant/1 -> Relational Operator/2
  Relational Operator/1 -> Logical Operator/2
  Logical Operator/1 -> Memory/1, Done/1, Switch1/2
  Memory/1 -> Logical Operator/1

== system firefighting_drone_2/Search for Fire/Seaerch-fire/Search4/Move Arm2/If Action Subsystem ==
  In1 : Inport
  Action Port : ActionPort  ActionPortLabel=if(u1 > 0)
  Out1 : Outport  VectorParamsAs1DForOutWhenUnconnected=off
  wires:
  In1/1 -> Out1/1

== system firefighting_drone_2/Search for Fire/Seaerch-fire/Search4/Move Arm2/If Action Subsystem1 ==
  In1 : Inport
  Action Port : ActionPort  ActionPortLabel=else
  Out1 : Outport  VectorParamsAs1DForOutWhenUnconnected=off
  wires:
  In1/1 -> Out1/1

== system firefighting_drone_2/Search for Fire/Seaerch-fire/Search4/Move Arm2/Subsystem ==
  Desired Angle : Inport
  Current Angle : Inport  Port=2
  Abs : Abs  SaturateOnIntegerOverflow=off
  Constant : Constant
  Logical Operator : Logic  Operator=OR  AllPortsSameDT=off  OutDataTypeStr=boolean
  Memory : Memory
  Relational Operator : RelationalOperator  Operator=<=  OutDataTypeStr=boolean  RndMeth=Simplest  InputSameDT=off
  Sum : Sum  Inputs=|+-
  Switch1 : Switch  Criteria=u2 > Threshold  SaturateOnIntegerOverflow=off  InputSameDT=off
  Out1 : Outport  VectorParamsAs1DForOutWhenUnconnected=off
  Done : Outport  Port=2  VectorParamsAs1DForOutWhenUnconnected=off
  wires:
  Switch1/1 -> Out1/1
  Desired Angle/1 -> Sum/1, Switch1/1
  Current Angle/1 -> Switch1/3, Sum/2
  Sum/1 -> Abs/1
  Abs/1 -> Relational Operator/1
  Constant/1 -> Relational Operator/2
  Relational Operator/1 -> Logical Operator/2
  Logical Operator/1 -> Memory/1, Done/1, Switch1/2
  Memory/1 -> Logical Operator/1

== system firefighting_drone_2/Search for Fire/Seaerch-fire/Search4/Move Arm3/If Action Subsystem ==
  In1 : Inport
  Action Port : ActionPort  ActionPortLabel=if(u1 > 0)
  Out1 : Outport  VectorParamsAs1DForOutWhenUnconnected=off
  wires:
  In1/1 -> Out1/1

== system firefighting_drone_2/Search for Fire/Seaerch-fire/Search4/Move Arm3/If Action Subsystem1 ==
  In1 : Inport
  Action Port : ActionPort  ActionPortLabel=else
  Out1 : Outport  VectorParamsAs1DForOutWhenUnconnected=off
  wires:
  In1/1 -> Out1/1

== system firefighting_drone_2/Search for Fire/Seaerch-fire/Search4/Move Arm3/Subsystem ==
  Desired Angle : Inport
  Current Angle : Inport  Port=2
  Abs : Abs  SaturateOnIntegerOverflow=off
  Constant : Constant
  Logical Operator : Logic  Operator=OR  AllPortsSameDT=off  OutDataTypeStr=boolean
  Memory : Memory
  Relational Operator : RelationalOperator  Operator=<=  OutDataTypeStr=boolean  RndMeth=Simplest  InputSameDT=off
  Sum : Sum  Inputs=|+-
  Switch1 : Switch  Criteria=u2 > Threshold  SaturateOnIntegerOverflow=off  InputSameDT=off
  Out1 : Outport  VectorParamsAs1DForOutWhenUnconnected=off
  Done : Outport  Port=2  VectorParamsAs1DForOutWhenUnconnected=off
  wires:
  Switch1/1 -> Out1/1
  Desired Angle/1 -> Sum/1, Switch1/1
  Current Angle/1 -> Switch1/3, Sum/2
  Sum/1 -> Abs/1
  Abs/1 -> Relational Operator/1
  Constant/1 -> Relational Operator/2
  Relational Operator/1 -> Logical Operator/2
  Logical Operator/1 -> Memory/1, Done/1, Switch1/2
  Memory/1 -> Logical Operator/1

== system firefighting_drone_2/Search for Fire/Seaerch-fire/Search5/Move Arm1/If Action Subsystem ==
  In1 : Inport
  Action Port : ActionPort  ActionPortLabel=if(u1 > 0)
  Out1 : Outport  VectorParamsAs1DForOutWhenUnconnected=off
  wires:
  In1/1 -> Out1/1

== system firefighting_drone_2/Search for Fire/Seaerch-fire/Search5/Move Arm1/If Action Subsystem1 ==
  In1 : Inport
  Action Port : ActionPort  ActionPortLabel=else
  Out1 : Outport  VectorParamsAs1DForOutWhenUnconnected=off
  wires:
  In1/1 -> Out1/1

== system firefighting_drone_2/Search for Fire/Seaerch-fire/Search5/Move Arm1/Subsystem ==
  Desired Angle : Inport
  Current Angle : Inport  Port=2
  Abs : Abs  SaturateOnIntegerOverflow=off
  Constant : Constant
  Logical Operator : Logic  Operator=OR  AllPortsSameDT=off  OutDataTypeStr=boolean
  Memory : Memory
  Relational Operator : RelationalOperator  Operator=<=  OutDataTypeStr=boolean  RndMeth=Simplest  InputSameDT=off
  Scope : Scope
  Scope1 : Scope
  Sum : Sum  Inputs=|+-
  Switch1 : Switch  Criteria=u2 > Threshold  SaturateOnIntegerOverflow=off  InputSameDT=off
  Out1 : Outport  VectorParamsAs1DForOutWhenUnconnected=off
  Done : Outport  Port=2  VectorParamsAs1DForOutWhenUnconnected=off
  wires:
  Switch1/1 -> Out1/1
  Desired Angle/1 -> Scope/1, Sum/1, Switch1/1
  Current Angle/1 -> Scope1/1, Switch1/3, Sum/2
  Sum/1 -> Abs/1
  Abs/1 -> Relational Operator/1
  Constant/1 -> Relational Operator/2
  Relational Operator/1 -> Logical Operator/2
  Logical Operator/1 -> Memory/1, Done/1, Switch1/2
  Memory/1 -> Logical Operator/1

== system firefighting_drone_2/Search for Fire/Seaerch-fire/Search5/Move Arm2/If Action Subsystem ==
  In1 : Inport
  Action Port : ActionPort  ActionPortLabel=if(u1 > 0)
  Out1 : Outport  VectorParamsAs1DForOutWhenUnconnected=off
  wires:
  In1/1 -> Out1/1

== system firefighting_drone_2/Search for Fire/Seaerch-fire/Search5/Move Arm2/If Action Subsystem1 ==
  In1 : Inport
  Action Port : ActionPort  ActionPortLabel=else
  Out1 : Outport  VectorParamsAs1DForOutWhenUnconnected=off
  wires:
  In1/1 -> Out1/1

== system firefighting_drone_2/Search for Fire/Seaerch-fire/Search5/Move Arm2/Subsystem ==
  Desired Angle : Inport
  Current Angle : Inport  Port=2
  Abs : Abs  SaturateOnIntegerOverflow=off
  Constant : Constant
  Logical Operator : Logic  Operator=OR  AllPortsSameDT=off  OutDataTypeStr=boolean
  Memory : Memory
  Relational Operator : RelationalOperator  Operator=<=  OutDataTypeStr=boolean  RndMeth=Simplest  InputSameDT=off
  Sum : Sum  Inputs=|+-
  Switch1 : Switch  Criteria=u2 > Threshold  SaturateOnIntegerOverflow=off  InputSameDT=off
  Out1 : Outport  VectorParamsAs1DForOutWhenUnconnected=off
  Done : Outport  Port=2  VectorParamsAs1DForOutWhenUnconnected=off
  wires:
  Switch1/1 -> Out1/1
  Desired Angle/1 -> Sum/1, Switch1/1
  Current Angle/1 -> Switch1/3, Sum/2
  Sum/1 -> Abs/1
  Abs/1 -> Relational Operator/1
  Constant/1 -> Relational Operator/2
  Relational Operator/1 -> Logical Operator/2
  Logical Operator/1 -> Memory/1, Done/1, Switch1/2
  Memory/1 -> Logical Operator/1

== system firefighting_drone_2/Search for Fire/Seaerch-fire/Search5/Move Arm3/If Action Subsystem ==
  In1 : Inport
  Action Port : ActionPort  ActionPortLabel=if(u1 > 0)
  Out1 : Outport  VectorParamsAs1DForOutWhenUnconnected=off
  wires:
  In1/1 -> Out1/1

== system firefighting_drone_2/Search for Fire/Seaerch-fire/Search5/Move Arm3/If Action Subsystem1 ==
  In1 : Inport
  Action Port : ActionPort  ActionPortLabel=else
  Out1 : Outport  VectorParamsAs1DForOutWhenUnconnected=off
  wires:
  In1/1 -> Out1/1
